simulink model "ccmodel"  (R2017a)
settings: Solver=ode45  StartTime=0.0  StopTime=120  RelTol=1e-3
values from neighbouring files (symbols this model uses):
  b = [1 -2 -3]    [Bode_plot.m]    (also in Bode_plot_real_pole.m = [1 30]; Real_pole_zero.m = [1 110 1000])
undefined symbols (not defined in the file or in its folder): m
settings Model: Creator=sansh  LastModifiedBy=sansh

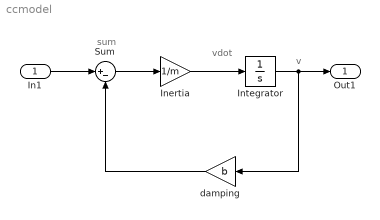
== system ccmodel ==
  note: v
  note: vdot
  note: sum
  In1 : Inport
  Inertia : Gain  Gain=1/m
  Integrator : Integrator
  Sum : Sum  Inputs=|+-
  damping : Gain  Gain=b
  Out1 : Outport
  wires:
  Integrator/1 -> Out1/1, damping/1
  Inertia/1 -> Integrator/1
  Sum/1 -> Inertia/1
  damping/1 -> Sum/2
  In1/1 -> Sum/1
